simulink model "TCU"  (R2016b)
settings: Solver=FixedStepAuto  StartTime=0  StopTime=inf  FixedStep=TCU.tiSimnTiStep_C  RelTol=1e-3  SampleTimeConstraint=STIndependent  EnableMultiTasking=on
settings Model: Creator=m01wolf  LastModifiedBy=bunver
settings DataIOCC: SaveFormat=StructureWithTime  SaveOutput=off  DSMLogging=off  VisualizeSimOutput=off  SaveTime=off  StateSaveName=Results  SignalLoggingName=Results
settings OptimizationCC: BlockReduction=off  ConditionallyExecuteInputs=off  LifeSpan=inf
settings DebuggingCC: AllowSymbolicDim=off  SFUnexpectedBacktrackingDiag=warning  SFNoUnconditionalDefaultTransitionDiag=warning  SFExecutionAtInitializationDiag=none
settings ModelReferenceCC: ModelReferenceNumInstancesAllowed=Single  PropagateSignalLabelsOutOfModel=off
settings GRTTargetCC: TargetLangStandard=C89/C90 (ANSI)
settings ConfigComp: CovMetricSettings=dw  CovHtmlReporting=on  CovSaveCumulativeToWorkspaceVar=on  CovSaveSingleToWorkspaceVar=on  CovExternalEMLEnable=off

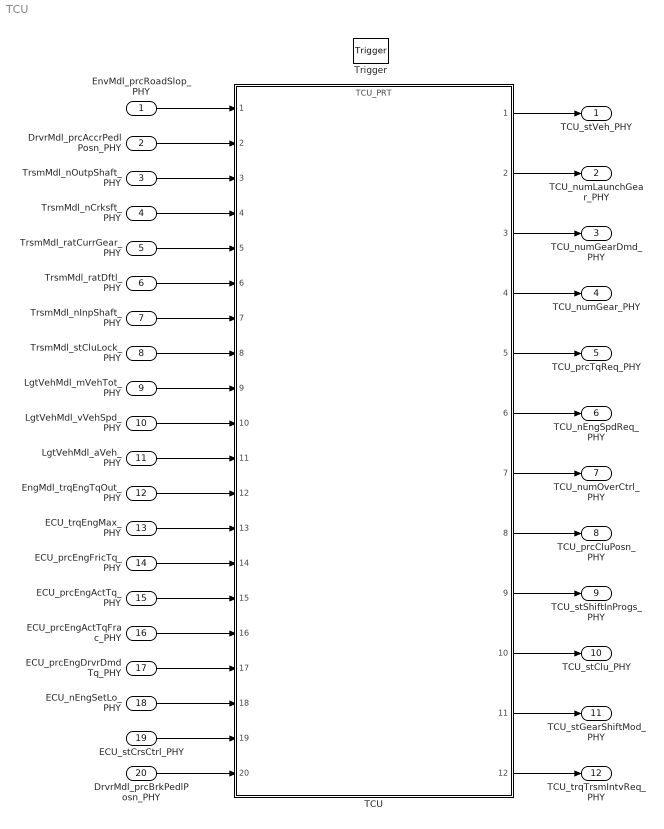
== system TCU ==
  EnvMdl_prcRoadSlop_PHY : Inport
  DrvrMdl_prcAccrPedlPosn_PHY : Inport  Port=2
  TrsmMdl_nOutpShaft_PHY : Inport  Port=3
  TrsmMdl_nCrksft_PHY : Inport  Port=4
  TrsmMdl_ratCurrGear_PHY : Inport  Port=5
  TrsmMdl_ratDftl_PHY : Inport  Port=6
  TrsmMdl_nInpShaft_PHY : Inport  Port=7
  TrsmMdl_stCluLock_PHY : Inport  Port=8
  LgtVehMdl_mVehTot_PHY : Inport  Port=9
  LgtVehMdl_vVehSpd_PHY : Inport  Port=10
  LgtVehMdl_aVeh_PHY : Inport  Port=11
  EngMdl_trqEngTqOut_PHY : Inport  Port=12
  ECU_trqEngMax_PHY : Inport  Port=13
  ECU_prcEngFricTq_PHY : Inport  Port=14
  ECU_prcEngActTq_PHY : Inport  Port=15
  ECU_prcEngActTqFrac_PHY : Inport  Port=16
  ECU_prcEngDrvrDmdTq_PHY : Inport  Port=17
  ECU_nEngSetLo_PHY : Inport  Port=18
  ECU_stCrsCtrl_PHY : Inport  Port=19
  DrvrMdl_prcBrkPedlPosn_PHY : Inport  Port=20
  Trigger : TriggerPort  TriggerType=function-call  VariantControl=Variant  PortDimensions=1
  TCU : ModelReference  ModelNameDialog=TCU_PRT.slxp  ModelReferenceVersion=1.262  CopyOfModelProtected=on
  TCU_stVeh_PHY : Outport
  TCU_numLaunchGear_PHY : Outport  Port=2
  TCU_numGearDmd_PHY : Outport  Port=3
  TCU_numGear_PHY : Outport  Port=4
  TCU_prcTqReq_PHY : Outport  Port=5
  TCU_nEngSpdReq_PHY : Outport  Port=6
  TCU_numOverCtrl_PHY : Outport  Port=7
  TCU_prcCluPosn_PHY : Outport  Port=8
  TCU_stShiftInProgs_PHY : Outport  Port=9
  TCU_stClu_PHY : Outport  Port=10
  TCU_stGearShiftMod_PHY : Outport  Port=11
  TCU_trqTrsmIntvReq_PHY : Outport  Port=12
  wires:
  EnvMdl_prcRoadSlop_PHY/1 -> TCU/1
  TrsmMdl_nOutpShaft_PHY/1 -> TCU/3
  DrvrMdl_prcAccrPedlPosn_PHY/1 -> TCU/2
  TrsmMdl_nCrksft_PHY/1 -> TCU/4
  TrsmMdl_ratCurrGear_PHY/1 -> TCU/5
  TrsmMdl_ratDftl_PHY/1 -> TCU/6
  TrsmMdl_nInpShaft_PHY/1 -> TCU/7
  TrsmMdl_stCluLock_PHY/1 -> TCU/8
  LgtVehMdl_mVehTot_PHY/1 -> TCU/9
  LgtVehMdl_vVehSpd_PHY/1 -> TCU/10
  LgtVehMdl_aVeh_PHY/1 -> TCU/11
  EngMdl_trqEngTqOut_PHY/1 -> TCU/12
  ECU_trqEngMax_PHY/1 -> TCU/13
  ECU_prcEngFricTq_PHY/1 -> TCU/14
  ECU_prcEngActTq_PHY/1 -> TCU/15
  ECU_prcEngActTqFrac_PHY/1 -> TCU/16
  ECU_prcEngDrvrDmdTq_PHY/1 -> TCU/17
  ECU_nEngSetLo_PHY/1 -> TCU/18
  TCU/1 -> TCU_stVeh_PHY/1
  TCU/2 -> TCU_numLaunchGear_PHY/1
  TCU/3 -> TCU_numGearDmd_PHY/1
  TCU/4 -> TCU_numGear_PHY/1
  TCU/5 -> TCU_prcTqReq_PHY/1
  TCU/6 -> TCU_nEngSpdReq_PHY/1
  TCU/7 -> TCU_numOverCtrl_PHY/1
  TCU/8 -> TCU_prcCluPosn_PHY/1
  TCU/9 -> TCU_stShiftInProgs_PHY/1
  TCU/10 -> TCU_stClu_PHY/1
  TCU/11 -> TCU_stGearShiftMod_PHY/1
  TCU/12 -> TCU_trqTrsmIntvReq_PHY/1
  ECU_stCrsCtrl_PHY/1 -> TCU/19
  DrvrMdl_prcBrkPedlPosn_PHY/1 -> TCU/20
